simulink model "TEST"  (R2018b)
settings: Solver=FixedStepAuto  StartTime=0.0  StopTime=20  FixedStep=1  RelTol=1e-3
PostLoadFcn:
  | if any(exist('dsrtsu_mdlpostloadfcn', 'file') ~= 0), dsrtsu_mdlpostloadfcn('Execute', bdroot); end
libraries: rtican x1
settings Model: DSRTSU_INTERNAL_RTI_VER=540  DSRTSU_INTERNAL_RTI_TYPE=rti1401  RTICANMMDATA=struct('GeneralSetupData',struct('modelroot','F:\src_cm4sl','generalsettings',struct('filesettings',struct('destfolder',struct('Name','RTICANMM_FILES','Check',1),'buildfolder',struct('Name','.','Check',1),'AbsDestfolder',struct('Name','F:\src_cm4sl\RTICANMM_FILES'),'AbsBuildfolder',struct('Name','F:\src_cm4sl'))),'options',struct('addpaths',1,'rmpaths',1,'addtrcexclusion',logical(1),'cannavigator',struct('checkmonitoring',0),'show_usrtrc',0,'use_usrtrc',0),'advanced',struct('options',ones(1,100)),'MPSetup',{{}},'RTI',struct('Type','GRT','Ver','','Date',''),'modelname','TEST','block','TEST'))  DSRTSU_INTERNAL_RTIFPGA=130  Creator=石丽  LastModifiedBy=石丽

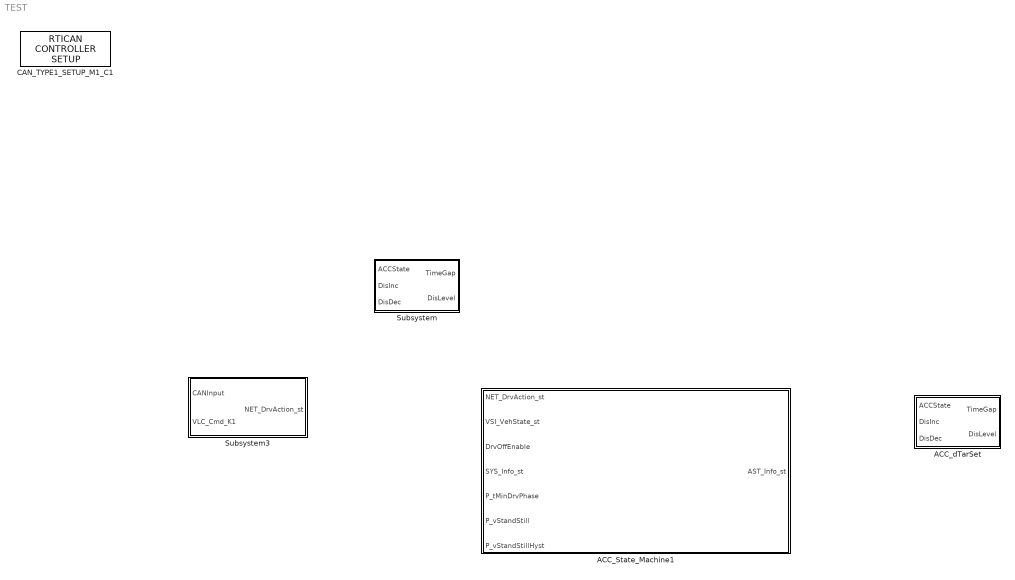
== system TEST ==
  ACC_State_Machine1 : Stateflow chart  TreatAsAtomicUnit=on
  ACC_dTarSet : Subsystem
  CAN_TYPE1_SETUP_M1_C1 : rtican/RTICAN CONTROLLER SETUP   Reserved1=[]  Reserved2=[]  Reserved3=[]  Reserved4=[]  AcceptanceMask=[]  ArbitrationField=[]  Parameters=[]  SFcnRTICANSettings=[]  MS_Struct=[]  BoardTypeNo=[]  BoardNo=[]  ChannelNo=[]  DialogFcn=[]  UnitName=[]  Revision=[]  UnitValues=[]  DSProperties=struct('RTI',struct('Version',uint32(12),'BlockType',struct('isSLSource',uint8(0),'isSLSink',uint8(0),'isHWSource',uint8(0),'isHWSink',uint8(0),'isSetup',uint8(1),'isInline',uint8(1),'isNonInline',uint8(0),'isInterrupt',uint8(0),'isChannelwise',uint8(0)),'IOBoardType','RTICAN','UnitType','NON_MESSAGE','Identifier','MASTER','DialogType','ML','BlockSet','RTICAN','SlaveProcessor','CAN'))  RTIBlockInterface=struct('InputPortsWidth',int32(0),'InputPortsActive',0,'OutputPortsWidth',int32(0),'OutputPortsActive',0,'DialogFcn','rtican_master_setup_gui','BlockDisplay',{{['CAN CONTROLLER\n SETUP'],'center'}},'IconTransparency','on','InitLevel',3,'IWork',{{{'',uint32(2)}}},'BlockName',struct('Token',{{'CAN_TYPE','_SETUP_M','_C'}},'BlockParam',{{'BoardTypeNo','BoardNo','ChannelNo'}}),'ParameterTunableNames',{{}})  RTIBlockParameters="struct('BoardTypeNo',{{1,'OFF',[]}},'BoardNo',{{1,'ON',[1 16]}},'ChannelNo',{{1,'ON',[1 2]}},'AcceptanceMask',{{0,'OFF',[]}},'ArbitrationField',{{0,'OFF',[]}},'Parameters',{{struct('Config',struct('Baudrate',500,'SampleMode',1,'UsedParamSet',1,'validSettings',1,'isBTRvalues',0,'Advanced',struct('Baudrate',{500,500,500},'Frequency',{24000000,36000000,64000000},'Settings',{struct('SMPL',0,'BRP',0,'NBT',24,'TSEG1',15,'TSEG2',6,'SJW',3,'SP',70),struct('SMPL',0,'BRP',1,'NBT',18,'TSEG1',14,'TSEG2',1,'SJW',1,'SP',88),struct('SMPL',0,'BRP',3,'NBT',16,'TSEG1',12,'TSEG2',1,'SJW',1,'SP',87)},'BTR0',{192,65,67},'BTR1',{111,30,28})),'configType',1,'Options',struct('DataFileSelected',1,'DataFileName',{{'dbc\\eyeq4_public.dbc'}},'DataFileDate',{{['09-12月-2020 08:51:51']}},'InterfaceFcn','rtican_dbc_file_parser','InterfaceFcnFileName','','LabelConfigType','volatile','AcceptanceMaskSelected',0,'MsgDataType','AllwaysDouble','NumType','hex','MaskType','STD','AcceptanceMask',0,'ArbitrationField',0,'UseMultipleMessageAccess',0),'RxReceiveStdOptions',struct('RxServiceStdEnabled',0,'RxServiceStdMsgIdent',1000,'RxServiceStdIdentNumType',1,'RxServiceStdIdentMask',0,'RxServiceStdMaskNumType',1,'RxServiceStdQueueSize',64),'RxReceiveXtdOptions',struct('RxServiceXtdEnabled',0,'RxServiceXtdMsgIdent',1001,'RxServiceXtdIdentNumType',1,'RxServiceXtdIdentMask',0,'RxServiceXtdMaskNumType',1,'RxServiceXtdQueueSize',64),'PartialNetworkingOptions',struct('switchedon',0,'format',1,'idmask',['    XXXXX XXXXXXXX XXXXXXXX XXXXXXXX'],'idcode','0','idfilter','0','datamaskused',0,'datalength',1,'datamask','0x0000000000000000','partialnetworkenable',0),'general',struct('Termination_common',1,'Termination_C252',1,'BusConfigurationRegister',0,'Transceiver','ISO11898','isFromLib',0)),'OFF',[]}},'CCPParameters',{{struct('CRO',struct('Format','STD','NumFormat','hex','Id',1639),'DTO',struct('Format','STD','NumFormat','hex','Id',2017),'StationAdr',struct('NumFormat','hex','Value',57),'StationId',struct('Value',['dSPACE CCP Service']),'Enabled',0),'OFF',[]}},'XCPParameters',{{struct('MASTER',struct('Format','STD','NumFormat','hex','Id',256),'SLAVE',struct('Format','STD','NumFormat','hex','Id',510),'Enabled',0,'PIDTransmissionEnabled',0),'OFF',[]}},'GroupId',{{struct('Group',{{'RTICAN'}},'No',1,'Behavior',{{'EVER'}},'BlockType',{{'SOURCE'}},'NameChangeFlag',1),'OFF',[]}},'SFcnRTICANSettings',{{struct('Baudrate',500,'configType',1,'AdvancedConfig',struct('Frequency',{},'BTR0',{},'BTR1',{}),'UsedParamSet',1,'STDMaskSelected','no','XTDMaskSelected','no','BoardType','DS1','BoardNo',1,'ControllerNo',1,'Transceiver','ISO11898','BusConfigRegister',0,'TerminationRes',120,'UseMultipleMessageAccess','no','STDRXSrvcUsed','no','STDRXSrvcMsgId',1000,'STDRXSrvcMsgMask',0,'STDRXSrvcQueueSize',64,'XTDRXSrvcUsed','no','XTDRXSrvcMsgId',1001,'XTDRXSrvcQueueSize',64,'XTDRXSrvcMsgMask',0,'PN_IsPNTransciever',0,'PN_IsPNEnabled',0,'PN_MsgFormat',1,'PN_idcode',0,'PN_idmask',2047,'PN_datamaskused',0,'PN_datalength',0,'PN_datamask',['0xFF, 0xFF, 0xFF, 0xFF, 0xFF, 0xFF, 0xFF, 0xFF']),'OFF',[]}},'SFcnRTICCPSettings',{{struct('CRO',struct('Format','STD','NumFormat','hex','Id',1639),'DTO',struct('Format','STD','NumFormat','hex','Id',2017),'StationAdr',struct('NumFormat','hex','Value',57),'StationId',struct('Value',['dSPACE CCP Service']),'Enabled',0),'OFF',[]}},'SFcnRTIXCPSettings',{{struct('MASTER',struct('Format','STD','NumFormat','hex','Id',256),'SLAVE',struct('Format','STD','NumFormat','hex','Id',510),'Enabled',0,'PIDTransmissionEnabled',0),'OFF',[]}},'TLCFileName',{{'rtican_master_setup','OFF',[]}})"  RTISFcnParameters=struct('SFcnRTICANSettings','struct','SFcnRTICCPSettings','struct','SFcnRTIXCPSettings','struct','AcceptanceMask','int32','ArbitrationField','int32','TLCFileName','char')  RTIBlockParaDefault="struct('BoardTypeNo',4302,'BoardNo',1,'ChannelNo',1,'AcceptanceMask',0,'ArbitrationField',0,'Parameters',struct('Config',struct('Baudrate',500,'SampleMode',1,'UsedParamSet',1,'validSettings',1,'isBTRvalues',0,'Advanced',struct('Frequency',16000000,'BTR0',64,'BTR1',28,'Settings',struct('SMPL',0,'BRP',0,'NBT',16,'TSEG1',12,'TSEG2',1,'SJW',1,'SP',87))),'configType',1,'Options',struct('DataFileSelected',0,'DataFileName',{{['<no datafile support>']}},'DataFileDate',{{''}},'InterfaceFcn','rtican_dbc_file_parser','InterfaceFcnFileName','','LabelConfigType','volatile','AcceptanceMaskSelected',0,'MsgDataType','AllwaysDouble','NumType','hex','MaskType','STD','AcceptanceMask',0,'ArbitrationField',0,'UseMultipleMessageAccess',0),'RxReceiveStdOptions',struct('RxServiceStdEnabled',0,'RxServiceStdMsgIdent',1000,'RxServiceStdIdentNumType',1,'RxServiceStdIdentMask',0,'RxServiceStdMaskNumType',1,'RxServiceStdQueueSize',64),'RxReceiveXtdOptions',struct('RxServiceXtdEnabled',0,'RxServiceXtdMsgIdent',1001,'RxServiceXtdIdentNumType',1,'RxServiceXtdIdentMask',0,'RxServiceXtdMaskNumType',1,'RxServiceXtdQueueSize',64),'PartialNetworkingOptions',struct('switchedon',0,'format',1,'idmask',['    XXXXX XXXXXXXX XXXXXXXX XXXXXXXX'],'idcode','0','idfilter','0','datamaskused',0,'datalength',1,'datamask','0x0000000000000000','partialnetworkenable',0),'general',struct('Termination_common',1,'Termination_C252',1,'BusConfigurationRegister',0,'Transceiver','ISO11898','isFromLib',1)),'CCPParameters',struct('CRO',struct('Format','STD','NumFormat','hex','Id',1639),'DTO',struct('Format','STD','NumFormat','hex','Id',2017),'StationAdr',struct('NumFormat','hex','Value',57),'StationId',struct('Value',['dSPACE CCP Service']),'Enabled',0),'XCPParameters',struct('MASTER',struct('Format','STD','NumFormat','hex','Id',256),'SLAVE',struct('Format','STD','NumFormat','hex','Id',510),'Enabled',0,'PIDTransmissionEnabled',0),'GroupId',struct('Group',{{'RTICAN'}},'No',1,'Behavior',{{'EVER'}},'BlockType',{{'SOURCE'}},'NameChangeFlag',1),'SFcnRTICANSettings',struct('Baudrate',500,'configType',1,'AdvandedConfig',struct('Frequency',16000000,'BTR0','0x40','BTR1','0x1C'),'UsedParamSet',1,'STDMaskSelected','no','XTDMaskSelected','no','BoardType','DS4302','BoardNo',1,'ControllerNo',1,'Transceiver','ISO11898','BusConfigRegister',0,'TerminationRes',120,'UseMultipleMessageAccess','no','STDRXSrvcUsed','no','STDRXSrvcMsgId',1000,'STDRXSrvcMsgMask',0,'STDRXSrvcQueueSize',64,'XTDRXSrvcUsed','no','XTDRXSrvcMsgId',1001,'XTDRXSrvcQueueSize',64,'XTDRXSrvcMsgMask',0),'SFcnRTICCPSettings',struct('CRO',struct('Format','STD','NumFormat','hex','Id',1639),'DTO',struct('Format','STD','NumFormat','hex','Id',2017),'StationAdr',struct('NumFormat','hex','Value',57),'StationId',struct('Value',['dSPACE CCP Service']),'Enabled',0),'SFcnRTIXCPSettings',struct('MASTER',struct('Format','STD','NumFormat','hex','Id',256),'SLAVE',struct('Format','STD','NumFormat','hex','Id',510),'Enabled',0,'PIDTransmissionEnabled',0),'TLCFileName','rtican_master_setup')"
      settings: AttributesFormatString=Group Id: RTICAN1\n  SourceProductName=dSPACE RTI CAN Blockset
  Subsystem : Subsystem
  Subsystem3 : Subsystem

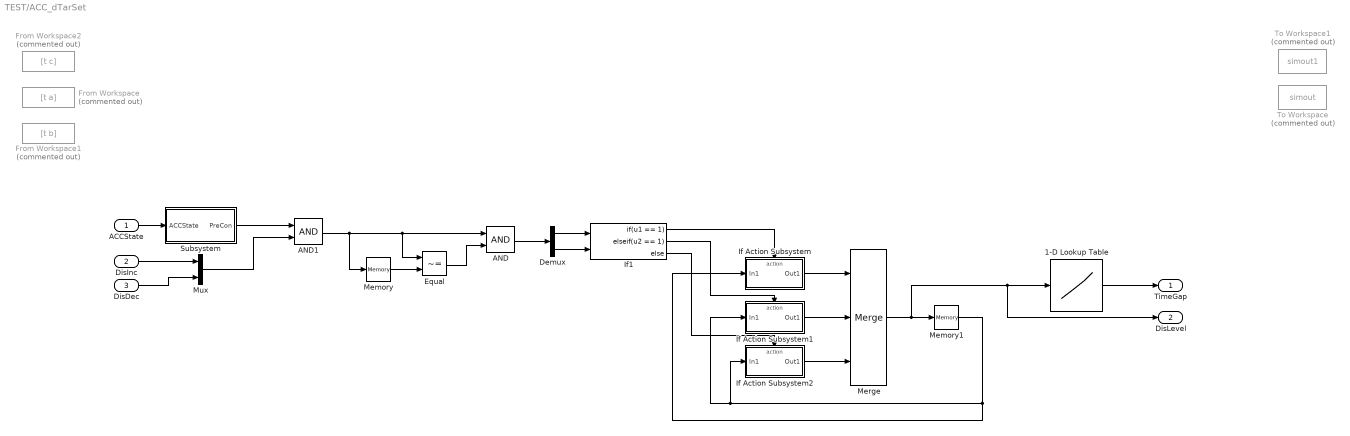
== system TEST/ACC_dTarSet ==
  ACCState : Inport
  DisInc : Inport  Port=2
  DisDec : Inport  Port=3
  1-D Lookup Table : Lookup_n-D  NumberOfTableDimensions=1  BreakpointsForDimension1=[1 2 3]  Table=[1.2 1.8 2.1]  InterpMethod=Flat  InternalRulePriority=Speed  RndMeth=Simplest  InputSameDT=on
  AND : Logic  AllPortsSameDT=off  OutDataTypeStr=boolean
  AND1 : Logic  AllPortsSameDT=off  OutDataTypeStr=boolean
  Demux : Demux  Outputs=2
  Equal : RelationalOperator  Operator=~=  OutDataTypeStr=boolean  RndMeth=Simplest
  From Workspace : FromWorkspace  Commented=on  VariableName=[t a]  SampleTime=0
  From Workspace1 : FromWorkspace  Commented=on  VariableName=[t b]  SampleTime=0
  From Workspace2 : FromWorkspace  Commented=on  VariableName=[t c]  SampleTime=0
  If Action Subsystem : Subsystem  TreatAsAtomicUnit=on
  If Action Subsystem1 : Subsystem  TreatAsAtomicUnit=on
  If Action Subsystem2 : Subsystem  TreatAsAtomicUnit=on
  If1 : If  NumInputs=2  IfExpression=u1 == 1  ElseIfExpressions=u2 == 1
  Memory : Memory
  Memory1 : Memory  InitialCondition=3
  Merge : Merge  Inputs=3  InitialOutput=0
  Mux : Mux  Inputs=2
  Subsystem : Subsystem
  To Workspace : ToWorkspace  Commented=on  VariableName=simout  SaveFormat=Timeseries  SampleTime=-1
  To Workspace1 : ToWorkspace  Commented=on  VariableName=simout1  SaveFormat=Timeseries  SampleTime=-1
  TimeGap : Outport
  DisLevel : Outport  Port=2
  wires:
  If1/1 -> If Action Subsystem/Action
  If Action Subsystem/1(Out1) -> Merge/1
  Memory1/1 -> If Action Subsystem/1(In1), If Action Subsystem1/1(In1), If Action Subsystem2/1(In1)
  If Action Subsystem1/1(Out1) -> Merge/2
  If1/2 -> If Action Subsystem1/Action
  If Action Subsystem2/1(Out1) -> Merge/3
  If1/3 -> If Action Subsystem2/Action
  Merge/1 -> DisLevel/1, 1-D Lookup Table/1, Memory1/1
  Subsystem/1(PreCon) -> AND1/1
  AND1/1 -> Memory/1, Equal/1, AND/1
  Memory/1 -> Equal/2
  Equal/1 -> AND/2
  AND/1 -> Demux/1
  Demux/1 -> If1/1
  Demux/2 -> If1/2
  Mux/1 -> AND1/2
  ACCState/1 -> Subsystem/1(ACCState)
  DisInc/1 -> Mux/1
  DisDec/1 -> Mux/2
  1-D Lookup Table/1 -> TimeGap/1

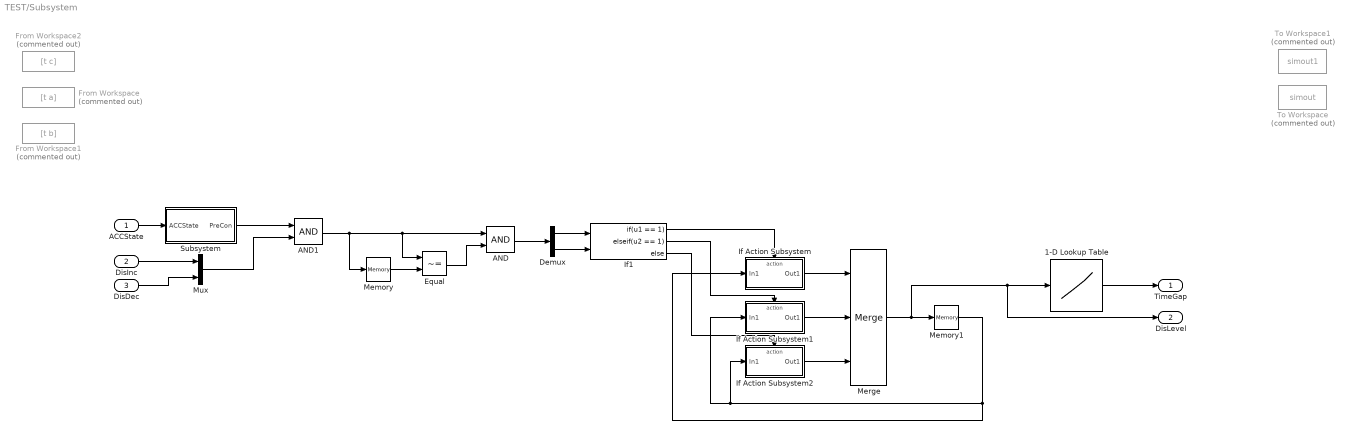
== system TEST/Subsystem ==
  ACCState : Inport
  DisInc : Inport  Port=2
  DisDec : Inport  Port=3
  1-D Lookup Table : Lookup_n-D  NumberOfTableDimensions=1  BreakpointsForDimension1=[1 2 3 4 5]  Table=[1.1 1.4 1.6 1.8 2.1]  InterpMethod=Flat  InternalRulePriority=Speed  RndMeth=Simplest  InputSameDT=on
  AND : Logic  AllPortsSameDT=off  OutDataTypeStr=boolean
  AND1 : Logic  AllPortsSameDT=off  OutDataTypeStr=boolean
  Demux : Demux  Outputs=2
  Equal : RelationalOperator  Operator=~=  OutDataTypeStr=boolean  RndMeth=Simplest
  From Workspace : FromWorkspace  Commented=on  VariableName=[t a]  SampleTime=0
  From Workspace1 : FromWorkspace  Commented=on  VariableName=[t b]  SampleTime=0
  From Workspace2 : FromWorkspace  Commented=on  VariableName=[t c]  SampleTime=0
  If Action Subsystem : Subsystem  TreatAsAtomicUnit=on
  If Action Subsystem1 : Subsystem  TreatAsAtomicUnit=on
  If Action Subsystem2 : Subsystem  TreatAsAtomicUnit=on
  If1 : If  NumInputs=2  IfExpression=u1 == 1  ElseIfExpressions=u2 == 1
  Memory : Memory
  Memory1 : Memory  InitialCondition=5
  Merge : Merge  Inputs=3  InitialOutput=0
  Mux : Mux  Inputs=2
  Subsystem : Subsystem
  To Workspace : ToWorkspace  Commented=on  VariableName=simout  SaveFormat=Timeseries  SampleTime=-1
  To Workspace1 : ToWorkspace  Commented=on  VariableName=simout1  SaveFormat=Timeseries  SampleTime=-1
  TimeGap : Outport
  DisLevel : Outport  Port=2
  wires:
  If1/1 -> If Action Subsystem/Action
  If Action Subsystem/1(Out1) -> Merge/1
  Memory1/1 -> If Action Subsystem/1(In1), If Action Subsystem1/1(In1), If Action Subsystem2/1(In1)
  If Action Subsystem1/1(Out1) -> Merge/2
  If1/2 -> If Action Subsystem1/Action
  If Action Subsystem2/1(Out1) -> Merge/3
  If1/3 -> If Action Subsystem2/Action
  Merge/1 -> DisLevel/1, 1-D Lookup Table/1, Memory1/1
  Subsystem/1(PreCon) -> AND1/1
  AND1/1 -> Memory/1, Equal/1, AND/1
  Memory/1 -> Equal/2
  Equal/1 -> AND/2
  AND/1 -> Demux/1
  Demux/1 -> If1/1
  Demux/2 -> If1/2
  Mux/1 -> AND1/2
  ACCState/1 -> Subsystem/1(ACCState)
  DisInc/1 -> Mux/1
  DisDec/1 -> Mux/2
  1-D Lookup Table/1 -> TimeGap/1

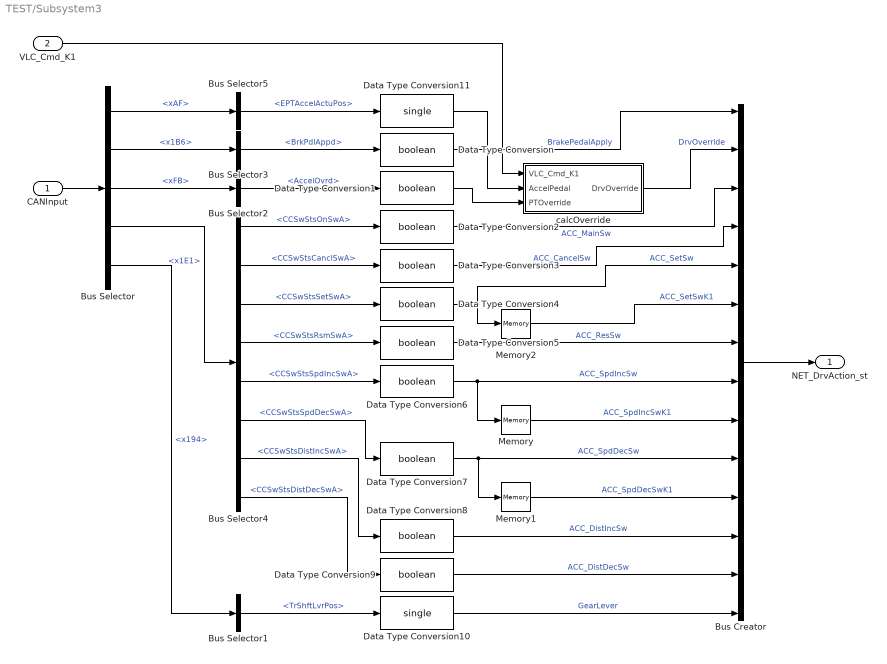
== system TEST/Subsystem3 ==
  CANInput : Inport
  VLC_Cmd_K1 : Inport  Port=2
  Bus Creator : BusCreator  Inputs=14  OutDataTypeStr=Bus: NET_DRVACTION_ST  NonVirtualBus=on
  Bus Selector : BusSelector  OutputSignals=xAF,x1B6,xFB,x1E1,x194
  Bus Selector1 : BusSelector  OutputSignals=TrShftLvrPos
  Bus Selector2 : BusSelector  OutputSignals=AccelOvrd
  Bus Selector3 : BusSelector  OutputSignals=BrkPdlAppd
  Bus Selector4 : BusSelector  OutputSignals=CCSwStsOnSwA,CCSwStsCanclSwA,CCSwStsSetSwA,CCSwStsRsmSwA,CCSwStsSpdIncSwA,CCSwStsSpdDecSwA,CCSwStsDistIncSwA,CCSwStsDistDecSwA
  Bus Selector5 : BusSelector  OutputSignals=EPTAccelActuPos
  Data Type Conversion{,1..9} (10 alike) : DataTypeConversion  OutDataTypeStr=boolean
  Data Type Conversion10 : DataTypeConversion  OutDataTypeStr=single
  Data Type Conversion11 : DataTypeConversion  OutDataTypeStr=single
  Memory : Memory
  Memory1 : Memory
  Memory2 : Memory
  calcOverride : Subsystem
  NET_DrvAction_st : Outport  OutDataTypeStr=Bus: NET_DRVACTION_ST
  wires:
  CANInput/1 -> Bus Selector/1
  Bus Selector/5 -> Bus Selector1/1  "<x194>"
  Bus Selector/3 -> Bus Selector2/1  "<xFB>"
  Bus Selector/2 -> Bus Selector3/1  "<x1B6>"
  Bus Selector/4 -> Bus Selector4/1  "<x1E1>"
  Bus Selector3/1 -> Data Type Conversion/1  "<BrkPdlAppd>"
  Data Type Conversion/1 -> Bus Creator/1  "BrakePedalApply"
  Bus Selector2/1 -> Data Type Conversion1/1  "<AccelOvrd>"
  Bus Selector4/1 -> Data Type Conversion2/1  "<CCSwStsOnSwA>"
  Bus Selector4/2 -> Data Type Conversion3/1  "<CCSwStsCanclSwA>"
  Bus Selector4/3 -> Data Type Conversion4/1  "<CCSwStsSetSwA>"
  Bus Selector4/4 -> Data Type Conversion5/1  "<CCSwStsRsmSwA>"
  Bus Selector4/5 -> Data Type Conversion6/1  "<CCSwStsSpdIncSwA>"
  Bus Selector4/6 -> Data Type Conversion7/1  "<CCSwStsSpdDecSwA>"
  Data Type Conversion6/1 -> Bus Creator/8, Memory/1  "ACC_SpdIncSw"
  Memory/1 -> Bus Creator/9  "ACC_SpdIncSwK1"
  Data Type Conversion7/1 -> Memory1/1, Bus Creator/10  "ACC_SpdDecSw"
  Memory1/1 -> Bus Creator/11  "ACC_SpdDecSwK1"
  Data Type Conversion8/1 -> Bus Creator/12  "ACC_DistIncSw"
  Bus Selector4/7 -> Data Type Conversion8/1  "<CCSwStsDistIncSwA>"
  Data Type Conversion9/1 -> Bus Creator/13  "ACC_DistDecSw"
  Bus Selector4/8 -> Data Type Conversion9/1  "<CCSwStsDistDecSwA>"
  Data Type Conversion2/1 -> Bus Creator/3  "ACC_MainSw"
  Data Type Conversion3/1 -> Bus Creator/4  "ACC_CancelSw"
  Data Type Conversion4/1 -> Memory2/1, Bus Creator/5  "ACC_SetSw"
  Data Type Conversion5/1 -> Bus Creator/7  "ACC_ResSw"
  Bus Creator/1 -> NET_DrvAction_st/1
  Data Type Conversion10/1 -> Bus Creator/14  "GearLever"
  Bus Selector1/1 -> Data Type Conversion10/1  "<TrShftLvrPos>"
  Bus Selector/1 -> Bus Selector5/1  "<xAF>"
  Bus Selector5/1 -> Data Type Conversion11/1  "<EPTAccelActuPos>"
  calcOverride/1(DrvOverride) -> Bus Creator/2  "DrvOverride"
  VLC_Cmd_K1/1 -> calcOverride/1(VLC_Cmd_K1)
  Data Type Conversion11/1 -> calcOverride/2(AccelPedal)
  Data Type Conversion1/1 -> calcOverride/3(PTOverride)
  Memory2/1 -> Bus Creator/6  "ACC_SetSwK1"

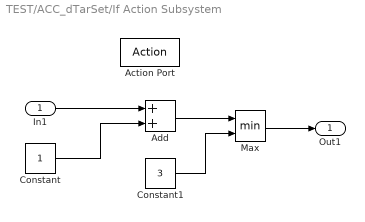
== system TEST/ACC_dTarSet/If Action Subsystem ==
  In1 : Inport
  Action Port : ActionPort
  Add : Sum
  Constant : Constant  OutDataTypeStr=single
  Constant1 : Constant  Value=3  OutDataTypeStr=single
  Max : MinMax  Inputs=2
  Out1 : Outport
  wires:
  In1/1 -> Add/1
  Constant/1 -> Add/2
  Max/1 -> Out1/1
  Add/1 -> Max/1
  Constant1/1 -> Max/2

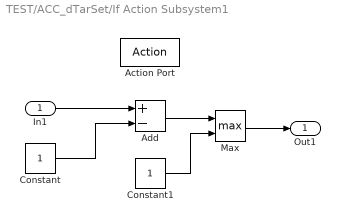
== system TEST/ACC_dTarSet/If Action Subsystem1 ==
  In1 : Inport
  Action Port : ActionPort
  Add : Sum  Inputs=+-
  Constant : Constant  OutDataTypeStr=single
  Constant1 : Constant  OutDataTypeStr=single
  Max : MinMax  Function=max  Inputs=2
  Out1 : Outport
  wires:
  In1/1 -> Add/1
  Constant/1 -> Add/2
  Add/1 -> Max/1
  Max/1 -> Out1/1
  Constant1/1 -> Max/2

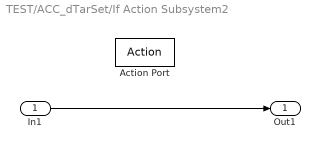
== system TEST/ACC_dTarSet/If Action Subsystem2 ==
  In1 : Inport
  Action Port : ActionPort
  Out1 : Outport
  wires:
  In1/1 -> Out1/1

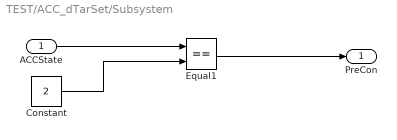
== system TEST/ACC_dTarSet/Subsystem ==
  ACCState : Inport
  Constant : Constant  Value=2  OutDataTypeStr=single
  Equal1 : RelationalOperator  Operator===  OutDataTypeStr=boolean  RndMeth=Simplest
  PreCon : Outport
  wires:
  Constant/1 -> Equal1/2
  ACCState/1 -> Equal1/1
  Equal1/1 -> PreCon/1

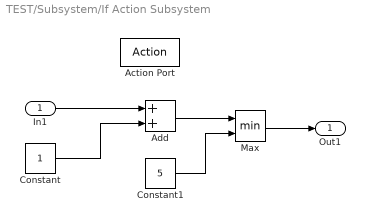
== system TEST/Subsystem/If Action Subsystem ==
  In1 : Inport
  Action Port : ActionPort  ActionType=then
  Add : Sum
  Constant : Constant  OutDataTypeStr=single
  Constant1 : Constant  Value=5  OutDataTypeStr=single
  Max : MinMax  Inputs=2
  Out1 : Outport
  wires:
  In1/1 -> Add/1
  Constant/1 -> Add/2
  Max/1 -> Out1/1
  Add/1 -> Max/1
  Constant1/1 -> Max/2

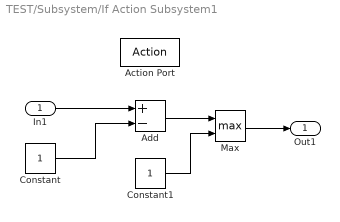
== system TEST/Subsystem/If Action Subsystem1 ==
  In1 : Inport
  Action Port : ActionPort  ActionType=elseif
  Add : Sum  Inputs=+-
  Constant : Constant  OutDataTypeStr=single
  Constant1 : Constant  OutDataTypeStr=single
  Max : MinMax  Function=max  Inputs=2
  Out1 : Outport
  wires:
  In1/1 -> Add/1
  Constant/1 -> Add/2
  Add/1 -> Max/1
  Max/1 -> Out1/1
  Constant1/1 -> Max/2

== system TEST/Subsystem/If Action Subsystem2 ==
  In1 : Inport
  Action Port : ActionPort  ActionType=else
  Out1 : Outport
  wires:
  In1/1 -> Out1/1

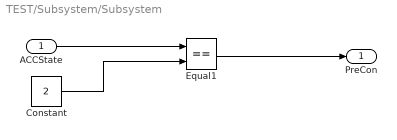
== system TEST/Subsystem/Subsystem ==
  ACCState : Inport
  Constant : Constant  Value=2  OutDataTypeStr=single
  Equal1 : RelationalOperator  Operator===  OutDataTypeStr=boolean  RndMeth=Simplest
  PreCon : Outport
  wires:
  Constant/1 -> Equal1/2
  ACCState/1 -> Equal1/1
  Equal1/1 -> PreCon/1

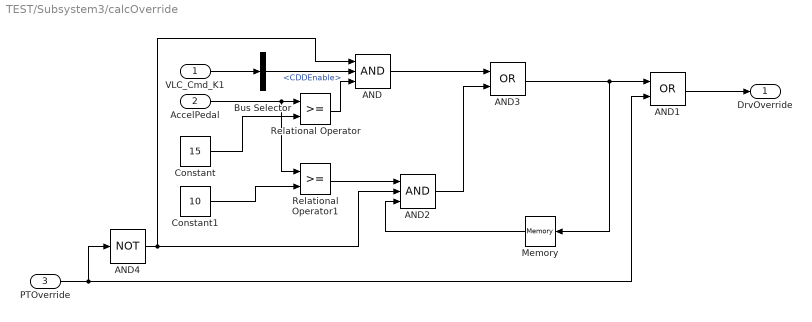
== system TEST/Subsystem3/calcOverride ==
  VLC_Cmd_K1 : Inport
  AccelPedal : Inport  Port=2
  PTOverride : Inport  Port=3
  AND : Logic  Inputs=3  AllPortsSameDT=off  OutDataTypeStr=boolean
  AND1 : Logic  Operator=OR  AllPortsSameDT=off  OutDataTypeStr=boolean
  AND2 : Logic  Inputs=3  AllPortsSameDT=off  OutDataTypeStr=boolean
  AND3 : Logic  Operator=OR  AllPortsSameDT=off  OutDataTypeStr=boolean
  AND4 : Logic  Operator=NOT  AllPortsSameDT=off  OutDataTypeStr=boolean
  Bus Selector : BusSelector  OutputSignals=CDDEnable
  Constant : Constant  Value=15
  Constant1 : Constant  Value=10
  Memory : Memory
  Relational Operator : RelationalOperator  OutDataTypeStr=boolean  RndMeth=Simplest
  Relational Operator1 : RelationalOperator  OutDataTypeStr=boolean  RndMeth=Simplest
  DrvOverride : Outport
  wires:
  VLC_Cmd_K1/1 -> Bus Selector/1
  AccelPedal/1 -> Relational Operator1/1, Relational Operator/1
  Constant/1 -> Relational Operator/2
  Bus Selector/1 -> AND/2  "<CDDEnable>"
  Relational Operator/1 -> AND/3
  AND3/1 -> AND1/1, Memory/1
  PTOverride/1 -> AND4/1, AND1/2
  AND1/1 -> DrvOverride/1
  Memory/1 -> AND2/3
  AND/1 -> AND3/1
  AND2/1 -> AND3/2
  Constant1/1 -> Relational Operator1/2
  Relational Operator1/1 -> AND2/1
  AND4/1 -> AND2/2, AND/1

== stateflow chart TEST/ACC_State_Machine1 ==
  note: MainState
      | 0	OFF
      | 1	PASSIVE
      | 2	ACTIVE_Drive
      | 3	ACTIVE_Standstill
      | 4	OVERRIDE
  state OFF
    en:
    AST_Info_st.MainState = 0;
    AST_Info_st.tMinInDrv = 0;
    AST_Info_st.vSet = 0;
  state OVERRIDE
    en:
    AST_Info_st.MainState = 4;
    AST_Info_st.tMinInDrv = 0;
  state PASSIVE
    en:
    AST_Info_st.MainState = 1;
    AST_Info_st.tMinInDrv = 0;
  state ACTIVE
    en:
    if ((NET_DrvAction_st.ACC_SetSw == 1)&&(NET_DrvAction_st.ACC_SetSwK1 == 0))
    AST_Info_st.vSet = VSI_VehState_st.vRef/1.05;
    end
    du:
    if ((NET_DrvAction_st.ACC_SpdIncSw == 1)&&(NET_DrvAction_st.ACC_SpdIncSwK1 == 0))
    AST_Info_st.vSet = floor(AST_Info_st.vSet*1.05*3.6)/1.05/3.6 + single(5 - mod(floor(AST_Info_st.vSet*1.05*3.6),5))/1.05/3.6;
    else if ((NET_DrvAction_st.ACC_SpdDecSw == 1)&&(NET_DrvAction_st.ACC_SpdDecSwK1 == 0))
    AST_Info_st.vSet = floor(AST_Info_st.vSet*1.05*3.6)/1.05/3.6 + single(mod(5 - mod(floor(AST_Info_st.vSet*1.05*3.6),5),5))/1.05/3.6 - 5/1.05/3.6;
    end
    end
    AST_Info_st.vSet = min(AST_Info_st.vSet, (120/1.05)/3.6);
    AST_Info_st.vSet = max(AST_Info_st.vSet, (30/1.05)/3.6);
    state Drive
      en:
      AST_Info_st.MainState = 2;
      du:
      if(VSI_VehState_st.vRef > P_vStandStillHyst)
      if(AST_Info_st.tMinInDrv > SYS_Info_st.dT)
      AST_Info_st.tMinInDrv = AST_Info_st.tMinInDrv - SYS_Info_st.dT;
      else
      AST_Info_st.tMinInDrv = 0;
      end
      end
    state Standstill
      en:
      AST_Info_st.MainState = 3;
      AST_Info_st.tMinInDrv = P_tMinDrvPhase;
    (default) -> Drive
    Drive -> Standstill : [VSI_VehState_st.vRef < P_vStandStill...
        | &&AST_Info_st.tMinInDrv == 0]
    Standstill -> Drive : [DrvOffEnable == 1]
  (default) -> OFF
  OVERRIDE -> OFF [order 3] : [NET_DrvAction_st.ACC_MainSw == 0]
  ACTIVE -> OFF [order 3] : [NET_DrvAction_st.ACC_MainSw == 0]
  OVERRIDE -> PASSIVE [order 2] : [NET_DrvAction_st.ACC_CancelSw == 1||NET_DrvAction_st.BrakePedalApply == 1||NET_DrvAction_st.GearLever < 3]
  ACTIVE -> OVERRIDE [order 1] : [NET_DrvAction_st.DrvOverride == 1]
  OVERRIDE -> ACTIVE [order 1] : [NET_DrvAction_st.DrvOverride == 0]
  OFF -> PASSIVE : [NET_DrvAction_st.ACC_MainSw == 1]
  PASSIVE -> OFF [order 2] : [NET_DrvAction_st.ACC_MainSw == 0]
  PASSIVE -> ACTIVE [order 1] : [(NET_DrvAction_st.ACC_SetSw == 1||(NET_DrvAction_st.ACC_ResSw == 1&&AST_Info_st.vSet ~= 0))&&NET_DrvAction_st.BrakePedalApply == 0&&NET_DrvAction_st.GearLever >= 3]
  ACTIVE -> PASSIVE [order 2] : [NET_DrvAction_st.ACC_CancelSw == 1||NET_DrvAction_st.BrakePedalApply == 1||NET_DrvAction_st.GearLever < 3]
  data: NET_DrvAction_st input; AST_Info_st output Bus: AST_INFO_ST; VSI_VehState_st input; DrvOffEnable input; SYS_Info_st input; P_tMinDrvPhase input; P_vStandStill input; P_vStandStillHyst input
